simulink model "simualzione_prova1"  (R2024b)
settings: Solver=ode1  StartTime=0.0  StopTime=10.0  FixedStep=0.001  RelTol=1e-3
values from neighbouring files (symbols this model uses):
  A = [-2, 1, 0; 0, -2, 0; 0, 0, -5]    [runme.m]
  B = [0; 1; -1]    [runme.m]
  C = eye(3)    [runme.m]
  D = zeros(3,1)    [runme.m]
  K = - place(A,B,[-10,-11,-9])    [runme.m]
settings Model: Creator=Lorenzo  LastModifiedBy=Lorenzo

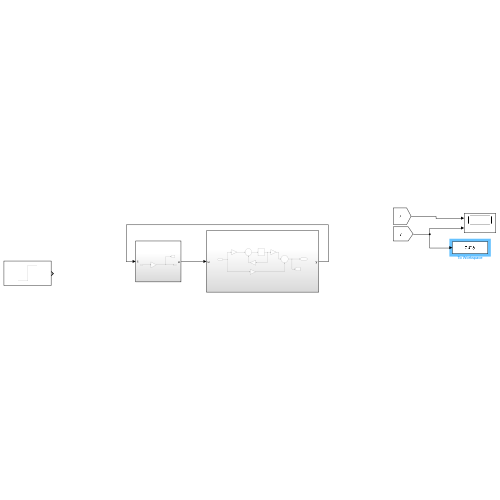
[thumbnail: Simulink's stored preview of the top-level diagram]
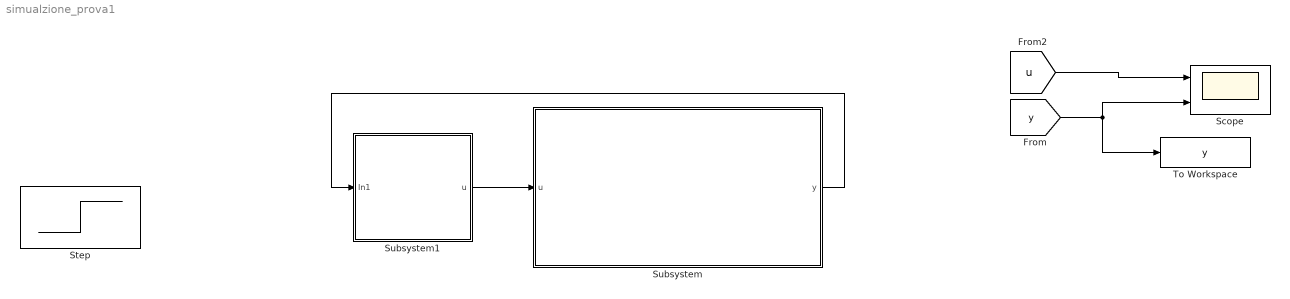
== system simualzione_prova1 ==
  Scope : Scope  NumInputPorts=2
  Step : Step  SampleTime=0
  Subsystem : Subsystem
  Subsystem1 : Subsystem
  To Workspace : ToWorkspace  VariableName=y  SaveFormat=Structure With Time  SampleTime=-1
  wires:
  [y] -> To Workspace/1, Scope/2
  [u] -> Scope/1
  Subsystem/1(y) -> Subsystem1/1(In1)
  Subsystem1/1(u) -> Subsystem/1(u)

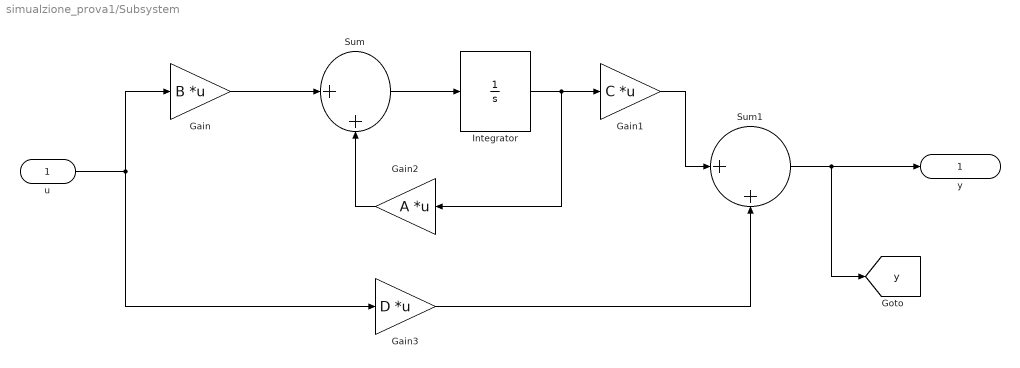
== system simualzione_prova1/Subsystem ==
  u : Inport
  Gain : Gain  Gain=B  Multiplication=Matrix(K*u)
  Gain1 : Gain  Gain=C  Multiplication=Matrix(K*u)
  Gain2 : Gain  Gain=A  Multiplication=Matrix(K*u)
  Gain3 : Gain  Gain=D  Multiplication=Matrix(K*u)
  Integrator : Integrator  InitialCondition=[1,2,3]
  Sum : Sum  Inputs=|++
  Sum1 : Sum  Inputs=|++
  y : Outport
  tag scope: y=global
  wires:
  Sum/1 -> Integrator/1
  Gain1/1 -> Sum1/1
  Gain3/1 -> Sum1/2
  Integrator/1 -> Gain2/1, Gain1/1
  u/1 -> Gain3/1, Gain/1
  Gain2/1 -> Sum/2
  Gain/1 -> Sum/1
  Sum1/1 -> [y], y/1

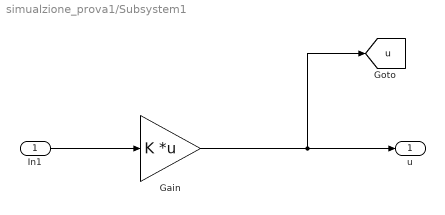
== system simualzione_prova1/Subsystem1 ==
  In1 : Inport
  Gain : Gain  Gain=K  Multiplication=Matrix(K*u)
  u : Outport
  tag scope: u=global
  wires:
  In1/1 -> Gain/1
  Gain/1 -> [u], u/1
